simulink library "color_detection_lib"  (R2025a)
settings: Solver=VariableStepAuto  StartTime=0.0  StopTime=10.0  RelTol=1e-3  EnableMultiTasking=on
undefined symbols (not defined in the file or in its folder): gcbh, xmcSameAsRefBlock
libraries: hlsBasic x6
settings Model: Creator=abehbood  LastModifiedBy=robg
settings SolverCC: AlgebraicLoopSolver=TrustRegion
settings DataIOCC: ReturnWorkspaceOutputs=off
settings OptimizationCC: LifeSpan=inf
settings DebuggingCC: UnconnectedInputMsg=warning  UnconnectedOutputMsg=warning  UnconnectedLineMsg=warning  SFUnexpectedBacktrackingDiag=warning  SFNoUnconditionalDefaultTransitionDiag=warning  ArithmeticOperatorsInVariantConditions=warning
settings ModelReferenceCC: EnableRefExpFcnMdlSchedulingChecks=on
settings SFSimCC: SimUseLocalCustomCode=off  CustomCodeUndefinedFunction=UseInterfaceOnly
settings RTWCC: RTWUseLocalCustomCode=off  GPUComputeCapability=3.5
settings CodeAppCC: StateflowObjectComments=on
settings GRTTargetCC: TargetLangStandard=C89/C90 (ANSI)
settings ConfigComp: CovMetricSettings=dw  CovSaveCumulativeToWorkspaceVar=on  CovSaveSingleToWorkspaceVar=on  CovExternalEMLEnable=off

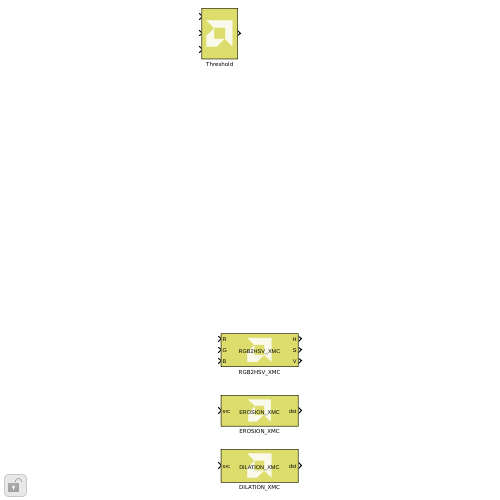
[thumbnail: Simulink's stored preview of the top-level diagram]
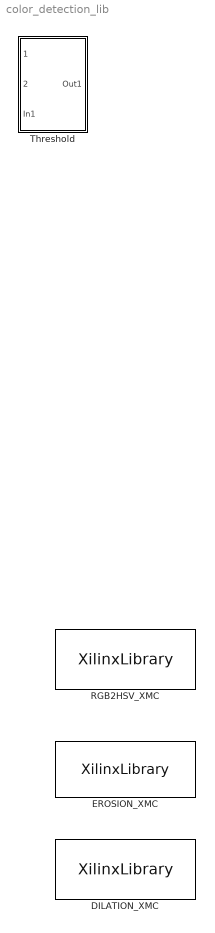
== system color_detection_lib ==
  DILATION_XMC : S-Function  InitFcn=xmcSameAsRefBlock(gcbh);  FunctionName=XilinxLibrary  Parameters=16 maskwsvariables  SFunctionDeploymentMode=off  EnableBusSupport=off  mask(Import Function){LibraryFunction=DILATION_XMC, IncludeFiles={'DILATION_wrap.h'}, SourceFiles={}, IncludeDirectories={'./include'}, TemplateParams={'int ROWS'; 'int COLS'}, FunctionParamTypes={xmcDataType('void'); xmcDataType('uint8_t'); xmcDataType('uint8_t'); xmcDataType('unsigned char')}, FunctionParamPassbys={0.000000000000000000e+00; 0.000000000000000000e+00; 0.000000000000000000e+00; 0.000000000000000000e+00}, FunctionParamDimensions={'1'; '[ROWS][COLS]'; '[ROWS][COLS]'; '[9]'}, FunctionParamNames={'return'; 'src'; 'dst'; 'kernel'}, FunctionParamDir={0.000000000000000000e+00; 1.000000000000000000e+00; 2.000000000000000000e+00; 3.000000000000000000e+00}, FunctionParamSupportsStreaming={true; true; true; true}, BufferDepth={'0'}, FunctionParamValues={'0'; '0'; '0'; '0'}, ThroughputFactors={''}, kernel=0}
      mask prompts: LibraryFunction "Function name:"; IncludeFiles "Main header file:"; SourceFiles "Source files:"; IncludeDirectories "Include directories:"; TemplateParams "Template parameters:"; FunctionParamTypes "Function parameter types:"; FunctionParamPassbys "Function parameter passbys:"; FunctionParamDimensions "Function parameter dimensions:"; FunctionParamNames "Function parameter names:"; FunctionParamDir "Function parameter directions:"; FunctionParamSupportsStreaming "Function parameter supports streaming:"; BufferDepth "Buffer depth:"; FunctionParamValues "Function parameter values:"; ThroughputFactors "Function throughput factors:"
      mask help: Function declaration<br><br>template&lt;int ROWS, int COLS&gt; void DILATION_XMC(uint8_t src[ROWS][COLS], uint8_t dst[ROWS][COLS], unsigned char kernel[9]);
      mask init:
      | maskwsvariables = get_param(gcbh,'maskwsvariables');
      | index_1 = find(strcmp({maskwsvariables.Name}, 'kernel') == 1);
      | value_1 = maskwsvariables(index_1).Value;
      | index = find(strcmp({maskwsvariables.Name}, 'FunctionParamValues') == 1);
      | maskwsvariables(index).Value = {'0'; '0'; '0'; xmcMatlab2CExp(value_1)};
      settings: PreCopyFcn=xmcWarnForDuplicateLibraryImportFunctionBlock()
      mask Help: helpview([xmcGetBlockHTMLPath 'libraryfunction.html']);
      mask DialogControl DescGroupVar Prompt: Import Function
      mask DialogControl FuncTab Prompt: Function
      mask DialogControl tpGroup0 Prompt: Template parameters
      mask DialogControl tpname_label0 Prompt: Name
      mask DialogControl tptype_label0 Prompt: Type
      mask DialogControl tpname_label_0_1 Prompt: ROWS
      mask DialogControl tptype_label_0_1 Prompt: int
      mask DialogControl tpname_label_0_2 Prompt: COLS
      mask DialogControl tptype_label_0_2 Prompt: int
      mask DialogControl interfaces_group0 Prompt: Interfaces
      mask DialogControl direction_label0 Prompt: Direction
      mask DialogControl name_label0 Prompt: Name
      mask DialogControl type_label0 Prompt: Type
      mask DialogControl dimension_label0 Prompt: Dimension
      mask DialogControl ifValue_label0_5 Prompt: Value
      mask DialogControl direction_label_0_2 Prompt: Input
      mask DialogControl name_label_0_2 Prompt: src
      mask DialogControl type_label_0_2 Prompt: uint8_t
      mask DialogControl dimension_label_0_2 Prompt: [ROWS][COLS]
      mask DialogControl direction_label_0_3 Prompt: Output
      mask DialogControl name_label_0_3 Prompt: dst
      mask DialogControl type_label_0_3 Prompt: uint8_t
      mask DialogControl dimension_label_0_3 Prompt: [ROWS][COLS]
      mask DialogControl direction_label_0_5 Prompt: Parameter
      mask DialogControl name_label_0_5 Prompt: kernel
      mask DialogControl type_label_0_5 Prompt: unsigned char
      mask DialogControl dimension_label_0_5 Prompt: [9]
      mask DialogControl FuncGenTab Prompt: General
      mask DialogControl parameters_group Prompt: Parameters
      mask DialogControl import_button Prompt: Import
      mask DialogControl advanced_parameters_group Prompt: Advanced parameters
      mask Display:
      | xmcDrawBlockIcon();
      | disp([strrep(LibraryFunction, '_', '\_')],'texmode','on');
      | port_label('input', 1, 'src');
      | port_label('output', 1, 'dst');
  EROSION_XMC : S-Function  InitFcn=xmcSameAsRefBlock(gcbh);  FunctionName=XilinxLibrary  Parameters=16 maskwsvariables  SFunctionDeploymentMode=off  EnableBusSupport=off  mask(Import Function){LibraryFunction=EROSION_XMC, IncludeFiles={'EROSION_wrap.h'}, SourceFiles={}, IncludeDirectories={'./include'}, TemplateParams={'int ROWS'; 'int COLS'}, FunctionParamTypes={xmcDataType('void'); xmcDataType('uint8_t'); xmcDataType('uint8_t'); xmcDataType('unsigned char')}, FunctionParamPassbys={0.000000000000000000e+00; 0.000000000000000000e+00; 0.000000000000000000e+00; 0.000000000000000000e+00}, FunctionParamDimensions={'1'; '[ROWS][COLS]'; '[ROWS][COLS]'; '[9]'}, FunctionParamNames={'return'; 'src'; 'dst'; 'kernel'}, FunctionParamDir={0.000000000000000000e+00; 1.000000000000000000e+00; 2.000000000000000000e+00; 3.000000000000000000e+00}, FunctionParamSupportsStreaming={true; true; true; true}, BufferDepth={'0'}, FunctionParamValues={'0'; '0'; '0'; '0'}, ThroughputFactors={''}, kernel=0}
      mask prompts: LibraryFunction "Function name:"; IncludeFiles "Main header file:"; SourceFiles "Source files:"; IncludeDirectories "Include directories:"; TemplateParams "Template parameters:"; FunctionParamTypes "Function parameter types:"; FunctionParamPassbys "Function parameter passbys:"; FunctionParamDimensions "Function parameter dimensions:"; FunctionParamNames "Function parameter names:"; FunctionParamDir "Function parameter directions:"; FunctionParamSupportsStreaming "Function parameter supports streaming:"; BufferDepth "Buffer depth:"; FunctionParamValues "Function parameter values:"; ThroughputFactors "Function throughput factors:"
      mask help: Function declaration<br><br>template&lt;int ROWS, int COLS&gt; void EROSION_XMC(uint8_t src[ROWS][COLS], uint8_t dst[ROWS][COLS], unsigned char kernel[9]);
      mask init: same as color_detection_lib/DILATION_XMC
      settings: PreCopyFcn=xmcWarnForDuplicateLibraryImportFunctionBlock()
      mask Help: helpview([xmcGetBlockHTMLPath 'libraryfunction.html']);
      mask DialogControl DescGroupVar Prompt: Import Function
      mask DialogControl FuncTab Prompt: Function
      mask DialogControl tpGroup0 Prompt: Template parameters
      mask DialogControl tpname_label0 Prompt: Name
      mask DialogControl tptype_label0 Prompt: Type
      mask DialogControl tpname_label_0_1 Prompt: ROWS
      mask DialogControl tptype_label_0_1 Prompt: int
      mask DialogControl tpname_label_0_2 Prompt: COLS
      mask DialogControl tptype_label_0_2 Prompt: int
      mask DialogControl interfaces_group0 Prompt: Interfaces
      mask DialogControl direction_label0 Prompt: Direction
      mask DialogControl name_label0 Prompt: Name
      mask DialogControl type_label0 Prompt: Type
      mask DialogControl dimension_label0 Prompt: Dimension
      mask DialogControl ifValue_label0_5 Prompt: Value
      mask DialogControl direction_label_0_2 Prompt: Input
      mask DialogControl name_label_0_2 Prompt: src
      mask DialogControl type_label_0_2 Prompt: uint8_t
      mask DialogControl dimension_label_0_2 Prompt: [ROWS][COLS]
      mask DialogControl direction_label_0_3 Prompt: Output
      mask DialogControl name_label_0_3 Prompt: dst
      mask DialogControl type_label_0_3 Prompt: uint8_t
      mask DialogControl dimension_label_0_3 Prompt: [ROWS][COLS]
      mask DialogControl direction_label_0_5 Prompt: Parameter
      mask DialogControl name_label_0_5 Prompt: kernel
      mask DialogControl type_label_0_5 Prompt: unsigned char
      mask DialogControl dimension_label_0_5 Prompt: [9]
      mask DialogControl FuncGenTab Prompt: General
      mask DialogControl parameters_group Prompt: Parameters
      mask DialogControl import_button Prompt: Import
      mask DialogControl advanced_parameters_group Prompt: Advanced parameters
      mask Display:
      | xmcDrawBlockIcon();
      | disp([strrep(LibraryFunction, '_', '\_')],'texmode','on');
      | port_label('input', 1, 'src');
      | port_label('output', 1, 'dst');
  RGB2HSV_XMC : S-Function  InitFcn=xmcSameAsRefBlock(gcbh);  FunctionName=XilinxLibrary  Parameters=16 maskwsvariables  SFunctionDeploymentMode=off  EnableBusSupport=off  mask(Import Function){LibraryFunction=RGB2HSV_XMC, IncludeFiles={'RGB2HSV_wrap.h'}, SourceFiles={}, IncludeDirectories={'./include'}, TemplateParams={'int ROWS'; 'int COLS'}, FunctionParamTypes={xmcDataType('void'); xmcDataType('uint8_t'); xmcDataType('uint8_t'); xmcDataType('uint8_t'); xmcDataType('uint8_t'); xmcDataType('uint8_t'); xmcDataType('uint8_t')}, FunctionParamPassbys={0.000000000000000000e+00; 0.000000000000000000e+00; 0.000000000000000000e+00; 0.000000000000000000e+00; 0.000000000000000000e+00; 0.000000000000000000e+00; 0.000000000000000000e+00}, FunctionParamDimensions={'1'; '[ROWS][COLS]'; '[ROWS][COLS]'; '[ROWS][COLS]'; '[ROWS][COLS]'; '[ROWS][COLS]'; '[ROWS][COLS]'}, FunctionParamNames={'return'; 'R'; 'G'; 'B'; 'H'; 'S'; 'V'}, FunctionParamDir={0.000000000000000000e+00; 1.000000000000000000e+00; 1.000000000000000000e+00; 1.000000000000000000e+00; 2.000000000000000000e+00; 2.000000000000000000e+00; 2.000000000000000000e+00}, FunctionParamSupportsStreaming={true; true; true; true; true; true; true}, BufferDepth={'0'}, FunctionParamValues={'0'; '0'; '0'; '0'; '0'; '0'; '0'}, ThroughputFactors={''}}
      mask prompts: LibraryFunction "Function name:"; IncludeFiles "Main header file:"; SourceFiles "Source files:"; IncludeDirectories "Include directories:"; TemplateParams "Template parameters:"; FunctionParamTypes "Function parameter types:"; FunctionParamPassbys "Function parameter passbys:"; FunctionParamDimensions "Function parameter dimensions:"; FunctionParamNames "Function parameter names:"; FunctionParamDir "Function parameter directions:"; FunctionParamSupportsStreaming "Function parameter supports streaming:"; BufferDepth "Buffer depth:"; FunctionParamValues "Function parameter values:"; ThroughputFactors "Function throughput factors:"
      mask help: Function declaration<br><br>template&lt;int ROWS, int COLS&gt; void RGB2HSV_XMC(uint8_t R[ROWS][COLS], uint8_t G[ROWS][COLS], uint8_t B[ROWS][COLS], uint8_t H[ROWS][COLS], uint8_t S[ROWS][COLS], uint8_t V[ROWS][COLS]);
      mask init:
      | maskwsvariables = get_param(gcbh,'maskwsvariables');
      settings: PreCopyFcn=xmcWarnForDuplicateLibraryImportFunctionBlock()
      mask Help: helpview([xmcGetBlockHTMLPath 'libraryfunction.html']);
      mask DialogControl DescGroupVar Prompt: Import Function
      mask DialogControl FuncTab Prompt: Function
      mask DialogControl tpGroup0 Prompt: Template parameters
      mask DialogControl tpname_label0 Prompt: Name
      mask DialogControl tptype_label0 Prompt: Type
      mask DialogControl tpname_label_0_1 Prompt: ROWS
      mask DialogControl tptype_label_0_1 Prompt: int
      mask DialogControl tpname_label_0_2 Prompt: COLS
      mask DialogControl tptype_label_0_2 Prompt: int
      mask DialogControl interfaces_group0 Prompt: Interfaces
      mask DialogControl direction_label0 Prompt: Direction
      mask DialogControl name_label0 Prompt: Name
      mask DialogControl type_label0 Prompt: Type
      mask DialogControl dimension_label0 Prompt: Dimension
      mask DialogControl direction_label_0_2 Prompt: Input
      mask DialogControl name_label_0_2 Prompt: R
      mask DialogControl type_label_0_2 Prompt: uint8_t
      mask DialogControl dimension_label_0_2 Prompt: [ROWS][COLS]
      mask DialogControl direction_label_0_3 Prompt: Input
      mask DialogControl name_label_0_3 Prompt: G
      mask DialogControl type_label_0_3 Prompt: uint8_t
      mask DialogControl dimension_label_0_3 Prompt: [ROWS][COLS]
      mask DialogControl direction_label_0_4 Prompt: Input
      mask DialogControl name_label_0_4 Prompt: B
      mask DialogControl type_label_0_4 Prompt: uint8_t
      mask DialogControl dimension_label_0_4 Prompt: [ROWS][COLS]
      mask DialogControl direction_label_0_5 Prompt: Output
      mask DialogControl name_label_0_5 Prompt: H
      mask DialogControl type_label_0_5 Prompt: uint8_t
      mask DialogControl dimension_label_0_5 Prompt: [ROWS][COLS]
      mask DialogControl direction_label_0_6 Prompt: Output
      mask DialogControl name_label_0_6 Prompt: S
      mask DialogControl type_label_0_6 Prompt: uint8_t
      mask DialogControl dimension_label_0_6 Prompt: [ROWS][COLS]
      mask DialogControl direction_label_0_7 Prompt: Output
      mask DialogControl name_label_0_7 Prompt: V
      mask DialogControl type_label_0_7 Prompt: uint8_t
      mask DialogControl dimension_label_0_7 Prompt: [ROWS][COLS]
      mask DialogControl FuncGenTab Prompt: General
      mask DialogControl parameters_group Prompt: Parameters
      mask DialogControl import_button Prompt: Import
      mask DialogControl advanced_parameters_group Prompt: Advanced parameters
      mask Display:
      | xmcDrawBlockIcon();
      | disp([strrep(LibraryFunction, '_', '\_')],'texmode','on');
      | port_label('input', 1, 'R');
      | port_label('input', 2, 'G');
      | port_label('input', 3, 'B');
      | port_label('output', 1, 'H');
      | port_label('output', 2, 'S');
      | port_label('output', 3, 'V');
  Threshold : Subsystem
      mask Display: xmcDrawBlockIcon();

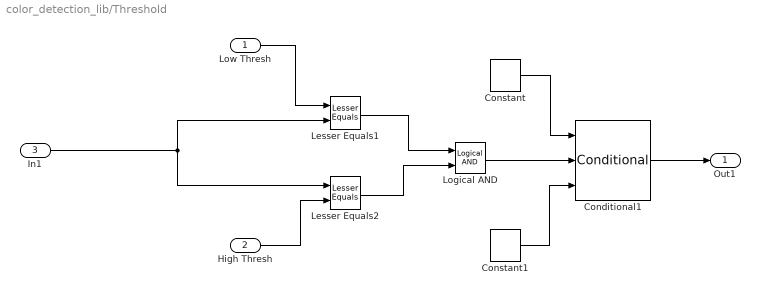
== system color_detection_lib/Threshold ==
  Low Thresh : Inport
  High Thresh : Inport  Port=2
  In1 : Inport  Port=3
  Conditional1 : hlsBasic/Conditional  Condition=C ~= 0  Threshold=0.00
  Constant : hlsBasic/Constant  Value=255  VectorParams1D=off  SampleTime=-1  OutDataType=uint8  TypeExp=''  Signedness=Signed  WordLength=16  FractionalLength=0  RoundingMode=Truncation to minus infinity  OverflowMode=Wrap around
  Constant1 : hlsBasic/Constant  Value=0  VectorParams1D=off  SampleTime=-1  OutDataType=uint8  TypeExp=''  Signedness=Signed  WordLength=16  FractionalLength=0  RoundingMode=Truncation to minus infinity  OverflowMode=Wrap around
  Lesser Equals1 : hlsBasic/Lesser Equals
  Lesser Equals2 : hlsBasic/Lesser Equals
  Logical AND : hlsBasic/Logical AND
  Out1 : Outport
  wires:
  Lesser Equals2/1 -> Logical AND/2
  Low Thresh/1 -> Lesser Equals1/1
  High Thresh/1 -> Lesser Equals2/2
  Lesser Equals1/1 -> Logical AND/1
  In1/1 -> Lesser Equals1/2, Lesser Equals2/1
  Logical AND/1 -> Conditional1/2
  Constant/1 -> Conditional1/1
  Constant1/1 -> Conditional1/3
  Conditional1/1 -> Out1/1
